simulink model "Physical_Model"  (R2024b)
settings: Solver=VariableStepAuto  StartTime=0.0  StopTime=10.0  RelTol=1e-3
values from neighbouring files (symbols this model uses):
  Fv_prime = Fv + 2*gbox.N^2*mot.Kt*mot.Ke/mot.R*[[1 -1];[-1 1]]    [MATRIX.m]
  g = 9.81    [balrob_params.m]
  g1 = 0    [MATRIX.m]
  M11 = 2 * wheel.Iyy + 2 * gbox.N^2 * mot.rot.Iyy + ( body.m + 2 * wheel.m + 2 * mot.rot.m ) * wheel.r^2    [MATRIX.m]
  M21 = M12    [MATRIX.m]
  M22 = body.Iyy + 2 * ( 1 - gbox.N )^2 * mot.rot.Iyy + body.m * body.zb^2 + 2 * mot.rot.m * mot.rot.zb^2    [MATRIX.m]
  ua2tau1 = ( 2 * gbox.N * mot.Kt / mot.R) * [1, -1]'    [MATRIX.m]
undefined symbols (not defined in the file or in its folder): body, mot, wheel
settings Model: Creator=fede  LastModifiedBy=Davide Pillon

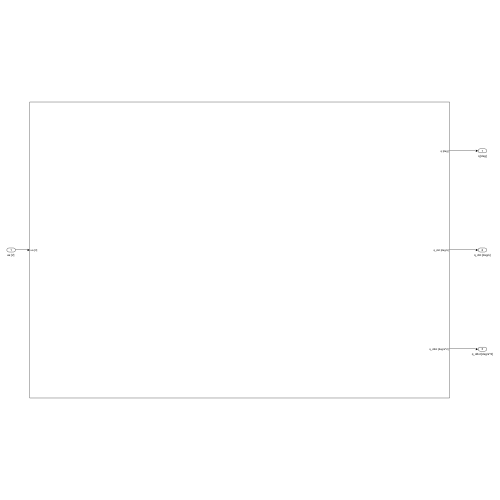
[thumbnail: Simulink's stored preview of the top-level diagram]
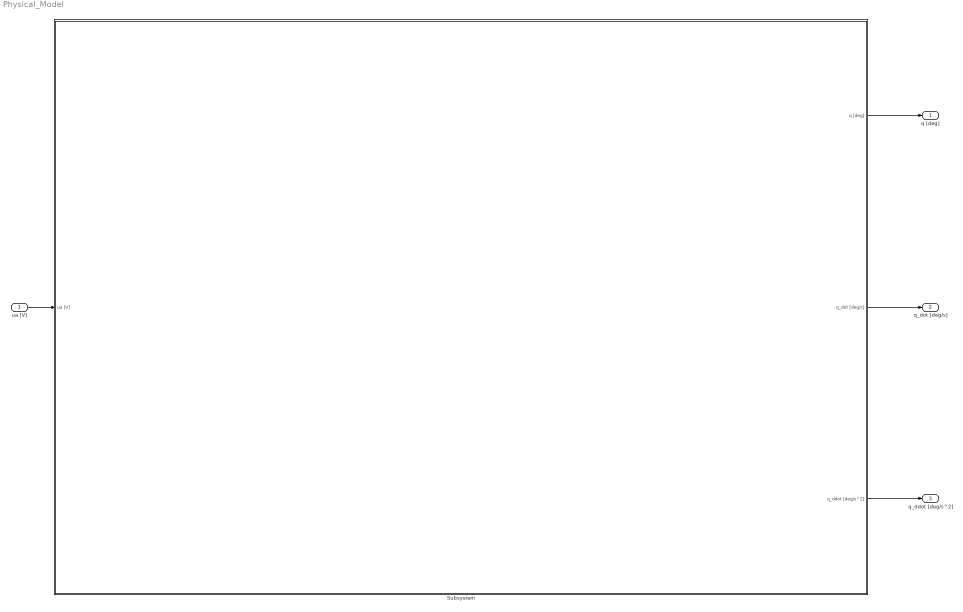
== system Physical_Model ==
  "ua [V] " : Inport
  Subsystem : Subsystem
  q [deg] : Outport
  q_dot [deg/s] : Outport  Port=2
  q_ddot [deg/s^2] : Outport  Port=3
  wires:
  "ua [V] "/1 -> Subsystem/1("ua [V] ")
  Subsystem/1(q [deg]) -> q [deg]/1
  Subsystem/2(q_dot [deg/s]) -> q_dot [deg/s]/1
  Subsystem/3(q_ddot [deg/s^2]) -> q_ddot [deg/s^2]/1

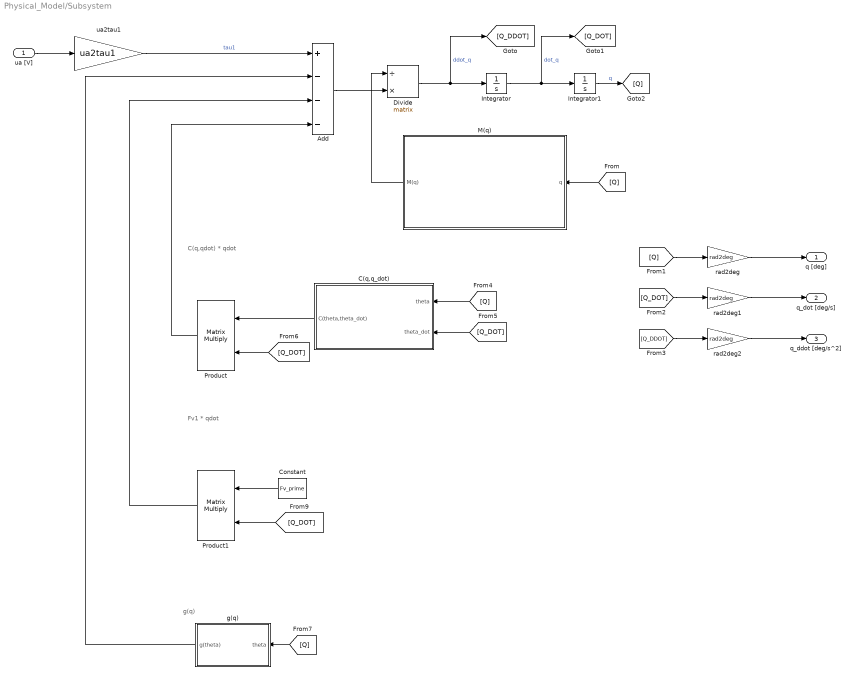
== system Physical_Model/Subsystem ==
  note: g(q)
  note: C(q,qdot) * qdot
  note: Fv1 * qdot
  "ua [V] " : Inport
  Add : Sum  Inputs=+---
  C(q,q_dot) : Subsystem
  Constant : Constant  Value=Fv_prime
  Divide : Product  Inputs=/*  Multiplication=Matrix(*)
  Integrator : Integrator
  Integrator1 : Integrator
  M(q) : Subsystem
  Product : Product  Multiplication=Matrix(*)
  Product1 : Product  Multiplication=Matrix(*)
  g(q) : Subsystem
  rad2deg : Gain  Gain=rad2deg
  rad2deg1 : Gain  Gain=rad2deg
  rad2deg2 : Gain  Gain=rad2deg
  ua2tau1 : Gain  Gain=ua2tau1
  q [deg] : Outport
  q_dot [deg/s] : Outport  Port=2
  q_ddot [deg/s^2] : Outport  Port=3
  wires:
  [Q_DOT] -> Product1/2
  [Q] -> M(q)/1(q)
  Divide/1 -> [Q_DDOT], Integrator/1  "ddot_q"
  Product/1 -> Add/4
  rad2deg/1 -> q [deg]/1
  [Q_DOT] -> Product/2
  g(q)/1(g(theta)) -> Add/2
  [Q_DOT] -> C(q,q_dot)/2(theta_dot)
  ua2tau1/1 -> Add/1  "tau1"
  [Q_DOT] -> rad2deg1/1
  Constant/1 -> Product1/1
  Integrator1/1 -> [Q]  "q"
  Integrator/1 -> [Q_DOT], Integrator1/1  "dot_q"
  [Q] -> rad2deg/1
  [Q] -> C(q,q_dot)/1(theta)
  "ua [V] "/1 -> ua2tau1/1
  Add/1 -> Divide/2
  Product1/1 -> Add/3
  [Q_DDOT] -> rad2deg2/1
  rad2deg2/1 -> q_ddot [deg/s^2]/1
  M(q)/1(M(q)) -> Divide/1
  [Q] -> g(q)/1(theta)
  C(q,q_dot)/1(C(theta,theta_dot)) -> Product/1
  rad2deg1/1 -> q_dot [deg/s]/1

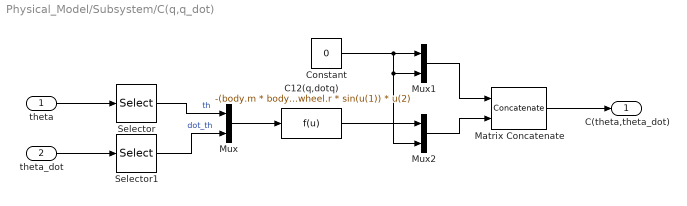
== system Physical_Model/Subsystem/C(q,q_dot) ==
  theta : Inport
  theta_dot : Inport  Port=2
  C12(q,dotq) : Fcn  Expr=-(body.m * body.zb + 2 * mot.rot.m * mot.rot.zb ) * wheel.r * sin(u(1)) * u(2)
  Constant : Constant  Value=0
  Matrix Concatenate : Concatenate  Mode=Multidimensional array  ConcatenateDimension=2
  Mux : Mux  Inputs=2
  Mux1 : Mux  Inputs=2
  Mux2 : Mux  Inputs=2
  Selector : Selector  InputPortWidth=2  IndexOptions=Index vector (dialog)  Indices=[2]  OutputSizes=1
  Selector1 : Selector  InputPortWidth=2  IndexOptions=Index vector (dialog)  Indices=[2]  OutputSizes=1
  C(theta,theta_dot) : Outport
  wires:
  Matrix Concatenate/1 -> C(theta,theta_dot)/1
  Mux2/1 -> Matrix Concatenate/2
  theta/1 -> Selector/1
  Constant/1 -> Mux2/2, Mux1/2, Mux1/1
  Mux/1 -> C12(q,dotq)/1
  Mux1/1 -> Matrix Concatenate/1
  Selector1/1 -> Mux/2  "dot_th"
  theta_dot/1 -> Selector1/1
  Selector/1 -> Mux/1  "th"
  C12(q,dotq)/1 -> Mux2/1

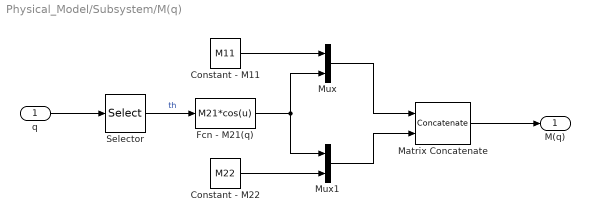
== system Physical_Model/Subsystem/M(q) ==
  q : Inport
  Constant - M11 : Constant  Value=M11
  Constant - M22 : Constant  Value=M22
  Fcn - M21(q) : Fcn  Expr=M21*cos(u)
  Matrix Concatenate : Concatenate  Mode=Multidimensional array  ConcatenateDimension=2
  Mux : Mux  Inputs=2
  Mux1 : Mux  Inputs=2
  Selector : Selector  InputPortWidth=2  IndexOptions=Index vector (dialog)  Indices=[2]  OutputSizes=1
  M(q) : Outport
  wires:
  Matrix Concatenate/1 -> M(q)/1
  Constant - M22/1 -> Mux1/2
  Fcn - M21(q)/1 -> Mux1/1, Mux/2
  q/1 -> Selector/1
  Mux/1 -> Matrix Concatenate/1
  Mux1/1 -> Matrix Concatenate/2
  Selector/1 -> Fcn - M21(q)/1  "th"
  Constant - M11/1 -> Mux/1

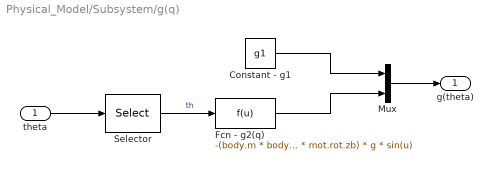
== system Physical_Model/Subsystem/g(q) ==
  theta : Inport
  Constant - g1 : Constant  Value=g1
  Fcn - g2(q) : Fcn  Expr=-(body.m * body.zb + 2 * mot.rot.m * mot.rot.zb) * g * sin(u)
  Mux : Mux  Inputs=2
  Selector : Selector  InputPortWidth=2  IndexOptions=Index vector (dialog)  Indices=[2]  OutputSizes=1
  g(theta) : Outport
  wires:
  Constant - g1/1 -> Mux/1
  Fcn - g2(q)/1 -> Mux/2
  Selector/1 -> Fcn - g2(q)/1  "th"
  theta/1 -> Selector/1
  Mux/1 -> g(theta)/1
